simulink model "openvf"  (R2024b)
settings: Solver=FixedStepDiscrete  StartTime=0.0  StopTime=1  FixedStep=1e-6  RelTol=1e-3
undefined symbols (not defined in the file): DiscIntNeverNeededParam
libraries: spsAsynchronousMachineSIUnitsLib x1, spsCurrentMeasurementLib x1, spsDCVoltageSourceLib x1, spsPWMGenerator2LevelLib x1, spsUniversalBridgeLib x1, spsVoltageMeasurementLib x1, sps_lib x1
settings Model: Creator=Ray  LastModifiedBy=suruchi raj
settings RTWCC: GPUComputeCapability=3.5

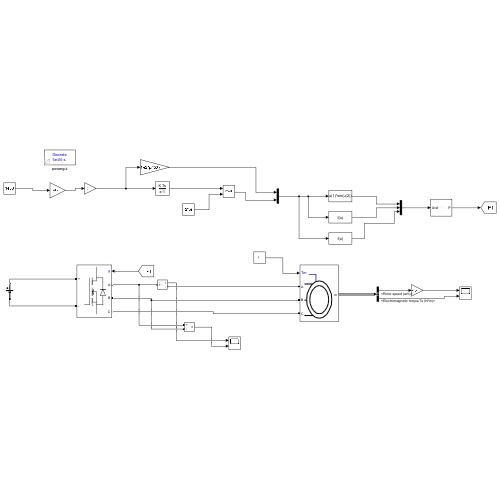
[thumbnail: Simulink's stored preview of the top-level diagram]
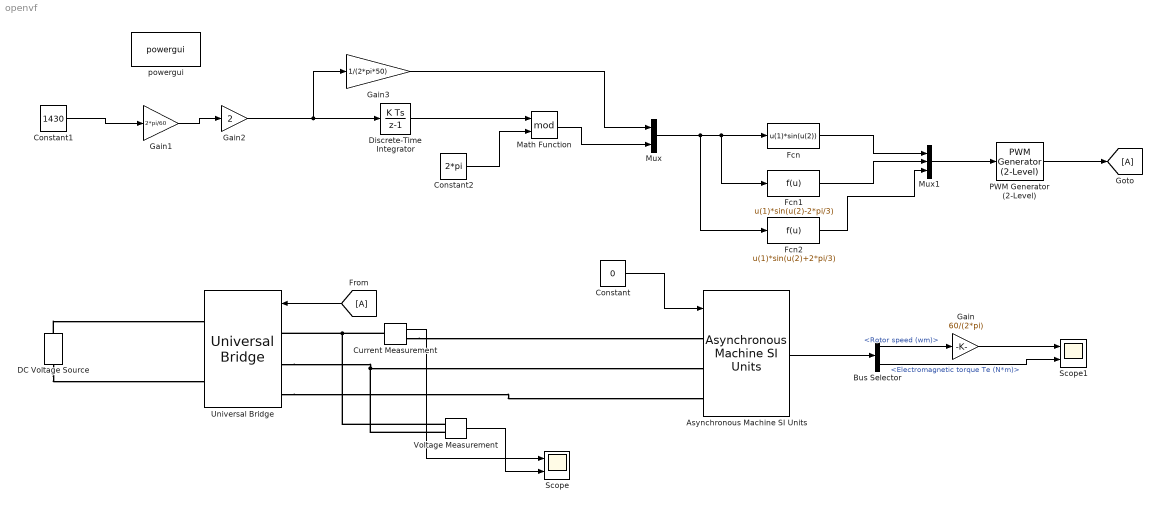
== system openvf ==
  Asynchronous Machine SI Units : spsAsynchronousMachineSIUnitsLib/Asynchronous Machine SI Units  RotorType=Squirrel-cage  PresetModel="15:  5.4 HP (4KW)   400 V  50Hz 1430 RPM"  MechanicalLoad=Torque Tm  ShowDetailedParameters=on  ReferenceFrame=Rotor  Units=SI  MeasurementBus=off  NominalParameters=[4000 400 50]  VoltageRatio=1  Stator=[1.405 0.005839]  Rotor=[1.395 0.005839]  Cage1=[0.4155 0.002066]  Cage2=[0.4168 0.0003495]  Lm=0.1722  Mechanical=[0.0131 0.002985 2]  PolePairs=2  InitialConditions=[0 0 0 0 0 0 0 0]  SimulateSaturation=off  Saturation=[14.03593122, 27.81365428, 53.79336849, 72.68890987, 97.98006896, 148.6815601, 215.7428561, 302.9841135, 428.7778367 ; 230, 322, 414, 460, 506, 552, 598, 644, 690]  LoadFlowParameters=1492000  TsPowergui=0  TsBlock=-1  IterativeModel=Trapezoidal non iterative  IterativeDiscreteModel=Trapezoidal non iterative  Pmec=1.492e+006
  Bus Selector : BusSelector  OutputSignals=Mechanical.Rotor speed (wm),Mechanical.Electromagnetic torque Te (N*m)
  Constant : Constant  Value=0
  Constant1 : Constant  Value=1430  SampleTime=50e-6
  Constant2 : Constant  Value=2*pi  SampleTime=50e-6
  Current Measurement : spsCurrentMeasurementLib/Current Measurement  PhasorSimulation=off  OutputType=Complex  PSBequivalent=0
  DC Voltage Source : spsDCVoltageSourceLib/DC Voltage Source  Amplitude=(400*sqrt(2)/sqrt(3))*2  Measurements=None
  Discrete-Time Integrator : DiscreteIntegrator  SampleTime=-1  ICPrevOutput=DiscIntNeverNeededParam  ICPrevScaledInput=DiscIntNeverNeededParam
  Fcn : Fcn  Expr=u(1)*sin(u(2))
  Fcn1 : Fcn  Expr=u(1)*sin(u(2)-2*pi/3)
  Fcn2 : Fcn  Expr=u(1)*sin(u(2)+2*pi/3)
  From : From
  Gain : Gain  Gain=60/(2*pi)
  Gain1 : Gain  Gain=2*pi/60
  Gain2 : Gain  Gain=2
  Gain3 : Gain  Gain=1/(2*pi*50)
  Goto : Goto
  Math Function : Math  Operator=mod
  Mux : Mux  Inputs=2
  Mux1 : Mux  Inputs=3
  PWM Generator (2-Level) : spsPWMGenerator2LevelLib/PWM Generator (2-Level)  ModulatorType=Three-phase bridge (6 pulses)  ModulatorMode=Unsynchronized  Fc=40*50  Pc=90  nF=27  MinMax="[ -1  1 ]"  SamplingTechnique=Natural  ModulatingSignals=off  m=0.8  Freq=60  Phase=0  Ts=50e-6  ShowCarrierOutport=off
  Scope : Scope  NumInputPorts=2
  Scope1 : Scope  NumInputPorts=2
  Universal Bridge : spsUniversalBridgeLib/Universal Bridge  Arms=3  SnubberResistance=1e5  SnubberCapacitance=inf  Device=MOSFET / Diodes  Ron=1e-3  Lon=0  ForwardVoltages="[  0  0  ]"  ForwardVoltage=0  GTOparameters=[ 10e-6 , 20e-6 ]  IGBTparameters=[ 1e-6 , 2e-6 ]  Measurements=None  Measurements_2=None  converterType=Rectifier
  Voltage Measurement : spsVoltageMeasurementLib/Voltage Measurement  PhasorSimulation=off  OutputType=Complex  PSBequivalent=0
  powergui : sps_lib/powergui  Priority=1  SimulationMode=Discrete  SampleTime=50e-6  frequency=60  Iterations=50  frequencyindice=50  Pbase=100e6  ErrMax=1e-4  UnitsV=kV  UnitsW=MW  buscounter=0  FunctionMessages=off  echomessages=off  EnableUseOfTLC=off  CurrentSourceSwitches=off  DisableSnubberDevices=off  DisableRonSwitches=off  DisableVfSwitches=off  DisplayEquations=off  AutomaticDiscreteSolvers=off  SolverType=Tustin/Backward Euler (TBE)  Interpol=off  ExternalGateDelay=off  methode=off  Ts=100  x0status=blocks  SPID=on  SwTol=0  HookPort=off  NonlinearTolerance=1e-4  nMaxIteration=100  ContinueOnMaxIteration=off  RestoreLinks=warning  ResistiveCurrentMeasurement=off  Frange=[0:2:500]  Ylog=off  Xlog=on  ShowGrid=off  save=off  variable=ZData  structure=0  ZoomFFT=off  StartTime=0.0  cycles=1  DisplayStyle=1  fundamental=60  FreqAxis=off  MaxFrequency=1000  frequencyindicesteady=1  RmsSteady=1  display=off
  wires:
  Current Measurement/1 -> Scope/1
  Voltage Measurement/1 -> Scope/2
  Asynchronous Machine SI Units/1 -> Bus Selector/1
  Bus Selector/1 -> Gain/1  "<Rotor speed (wm)>"
  Gain/1 -> Scope1/1
  Bus Selector/2 -> Scope1/2  "<Electromagnetic torque Te (N*m)>"
  Constant/1 -> Asynchronous Machine SI Units/1
  Constant1/1 -> Gain1/1
  Gain1/1 -> Gain2/1
  Gain2/1 -> Gain3/1, Discrete-Time Integrator/1
  Discrete-Time Integrator/1 -> Math Function/1
  Gain3/1 -> Mux/1
  Constant2/1 -> Math Function/2
  Math Function/1 -> Mux/2
  Mux/1 -> Fcn2/1, Fcn1/1, Fcn/1
  Fcn/1 -> Mux1/1
  Fcn1/1 -> Mux1/2
  Fcn2/1 -> Mux1/3
  Mux1/1 -> PWM Generator (2-Level)/1
  PWM Generator (2-Level)/1 -> Goto/1
  From/1 -> Universal Bridge/1
  connections:
  Current Measurement/LConn1 -- Voltage Measurement/LConn1 -- Universal Bridge/LConn1
  Current Measurement/RConn1 -- Asynchronous Machine SI Units/LConn1
  Universal Bridge/LConn2 -- Voltage Measurement/LConn2 -- Asynchronous Machine SI Units/LConn2
  Universal Bridge/LConn3 -- Asynchronous Machine SI Units/LConn3
  DC Voltage Source/RConn1 -- Universal Bridge/RConn1
  DC Voltage Source/LConn1 -- Universal Bridge/RConn2
